simulink model "shelf_cascade"  (R2024b)
settings: Solver=VariableStepAuto  StartTime=0.0  StopTime=10.0  RelTol=1e-3
libraries: dspsrcs4 x1
settings Model: Creator=woutlyen  LastModifiedBy=woutlyen

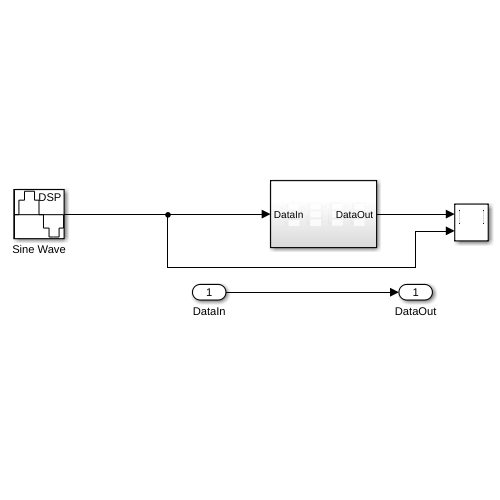
[thumbnail: Simulink's stored preview of the top-level diagram]
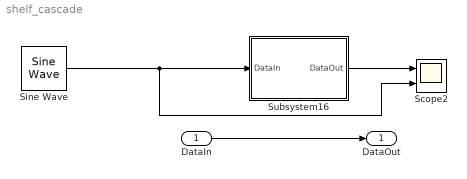
== system shelf_cascade ==
  DataIn : Inport  OutDataTypeStr=fixdt(1,24,23)
  Scope2 : Scope  NumInputPorts=2
  Sine Wave : dspsrcs4/Sine Wave  Amplitude=0.4467  Frequency=12000  Phase=0  SampleMode=Discrete  OutComplex=Real  CompMethod=Table lookup  TableSize=Speed  SampleTime=1/48000  SamplesPerFrame=1  ResetState=Restart at time zero  OutputFrames=off  dataType=Fixed-point  wordLen=24  udDataType=sfix(16)  fracBitsMode=User-defined  numFracBits=23  OutDataTypeStr=fixdt(1,24,23)  LastOutDataTypeStr=fixdt(1,24,23)
  Subsystem16 : Subsystem
  DataOut : Outport
  wires:
  Sine Wave/1 -> Subsystem16/1(DataIn), Scope2/2
  DataIn/1 -> DataOut/1
  Subsystem16/1(DataOut) -> Scope2/1

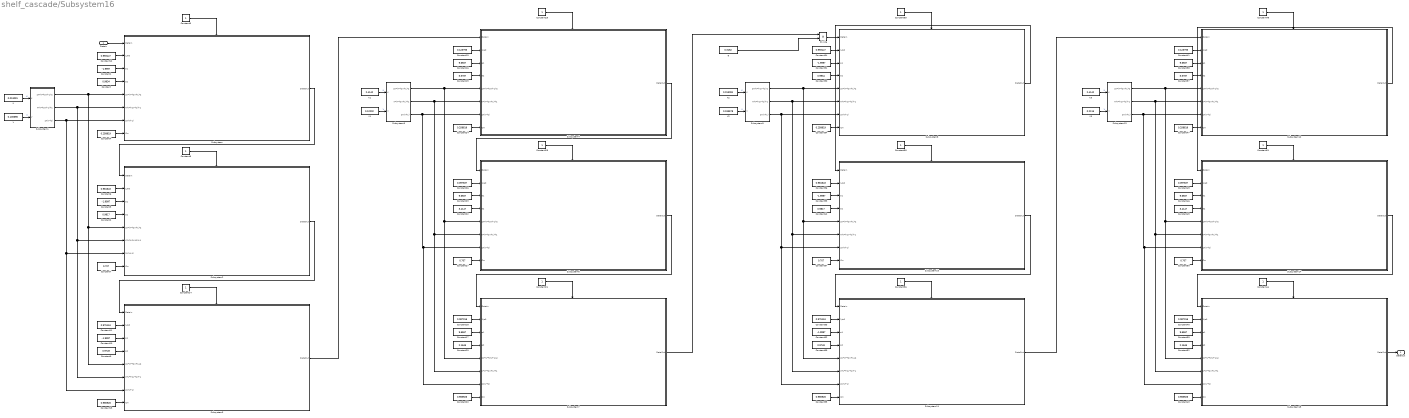
== system shelf_cascade/Subsystem16 ==
  DataIn : Inport
  Constant : Constant  Value=0.9934  OutDataTypeStr=fixdt(1,27,23)
  Constant{1,3,10,31..32,53} (6 alike) : Constant  Value=-1.9997  OutDataTypeStr=fixdt(1,27,23)
  Constant11 : Constant  Value=0.975134  OutDataTypeStr=fixdt(1,27,23)
  Constant12 : Constant  Value=0.993147  OutDataTypeStr=fixdt(1,27,23)
  Constant{13,20,35,43} (4 alike) : Constant  Value=0.965926  OutDataTypeStr=fixdt(1,27,23)
  Constant{5,8,14,21,25,28,36,44,48,51,55,58} (12 alike) : Constant  OutDataTypeStr=boolean
  Constant15 : Constant  Value=5.5787  OutDataTypeStr=fixdt(1,29,23)
  Constant{16..17,23,38..39,46} (6 alike) : Constant  Value=9.6567  OutDataTypeStr=fixdt(1,29,23)
  Constant18 : Constant  Value=0.087016  OutDataTypeStr=fixdt(1,29,23)
  Constant19 : Constant  Value=0.123793  OutDataTypeStr=fixdt(1,29,23)
  Constant2 : Constant  Value=0.9817  OutDataTypeStr=fixdt(1,27,23)
  Constant22 : Constant  Value=3.4147  OutDataTypeStr=fixdt(1,29,23)
  Constant{4,24,47,54} (4 alike) : Constant  Value=0.258819  OutDataTypeStr=fixdt(1,27,23)
  Constant26 : Constant  Value=0.097637  OutDataTypeStr=fixdt(1,29,23)
  Constant{7,27,50,57} (4 alike) : Constant  Value=0.707  OutDataTypeStr=fixdt(1,27,23)
  Constant29 : Constant  Value=2.1645  OutDataTypeStr=fixdt(1,29,23)
  Constant30 : Constant  Value=0.9934  OutDataTypeStr=fixdt(1,27,23)
  Constant33 : Constant  Value=0.975134  OutDataTypeStr=fixdt(1,27,23)
  Constant34 : Constant  Value=0.993147  OutDataTypeStr=fixdt(1,27,23)
  Constant37 : Constant  Value=5.5787  OutDataTypeStr=fixdt(1,29,23)
  Constant40 : Constant  Value=0.087016  OutDataTypeStr=fixdt(1,29,23)
  Constant41 : Constant  Value=0.123793  OutDataTypeStr=fixdt(1,29,23)
  Constant42 : Constant  Value=0.9817  OutDataTypeStr=fixdt(1,27,23)
  Constant45 : Constant  Value=3.4147  OutDataTypeStr=fixdt(1,29,23)
  Constant49 : Constant  Value=0.097637  OutDataTypeStr=fixdt(1,29,23)
  Constant52 : Constant  Value=2.1645  OutDataTypeStr=fixdt(1,29,23)
  Constant56 : Constant  Value=0.981643  OutDataTypeStr=fixdt(1,27,23)
  Constant59 : Constant  Value=0.9749  OutDataTypeStr=fixdt(1,27,23)
  Constant6 : Constant  Value=0.981643  OutDataTypeStr=fixdt(1,27,23)
  Constant9 : Constant  Value=0.9749  OutDataTypeStr=fixdt(1,27,23)
  Divide : Product  Inputs=**  OutDataTypeStr=fixdt(1,27,23)
  K : Constant  Value=0.013091  OutDataTypeStr=fixdt(1,27,23)
  K1 : Constant  Value=2.4142  OutDataTypeStr=fixdt(1,27,23)
  K2 : Constant  Value=0.013091  OutDataTypeStr=fixdt(1,27,23)
  K3 : Constant  Value=2.4142  OutDataTypeStr=fixdt(1,27,23)
  Subsystem : Subsystem
  Subsystem1 : Subsystem
  Subsystem10 : Subsystem
  Subsystem11 : Subsystem
  Subsystem12 : Subsystem
  Subsystem13 : Subsystem
  Subsystem14 : Subsystem
  Subsystem15 : Subsystem
  Subsystem2 : Subsystem
  Subsystem3 : Subsystem
  Subsystem4 : Subsystem
  Subsystem5 : Subsystem
  Subsystem6 : Subsystem
  Subsystem7 : Subsystem
  Subsystem8 : Subsystem
  Subsystem9 : Subsystem
  V : Constant  Value=0.100696  OutDataTypeStr=fixdt(1,27,23)
  V1 : Constant  Value=0.12202  OutDataTypeStr=fixdt(1,27,23)
  V2 : Constant  Value=0.193578  OutDataTypeStr=fixdt(1,27,23)
  V3 : Constant  Value=0.2115  OutDataTypeStr=fixdt(1,27,23)
  g : Constant  Value=0.3162  OutDataTypeStr=fixdt(1,27,23)
  DataOut : Outport
  wires:
  Subsystem2/1(DataOut) -> Subsystem3/1(DataIn)
  Constant7/1 -> Subsystem2/8(Cm)
  Constant21/1 -> Subsystem7/Enable
  Constant5/1 -> Subsystem/Enable
  V/1 -> Subsystem1/2(V)  "V"
  Constant48/1 -> Subsystem12/Enable
  Subsystem4/1(DataOut) -> Subsystem6/1(DataIn)
  Constant22/1 -> Subsystem6/4(a2)
  Constant16/1 -> Subsystem4/3(a1)
  Constant25/1 -> Subsystem4/Enable
  Subsystem7/1(DataOut) -> Divide/1
  Constant12/1 -> Subsystem/2(1/a0)
  V2/1 -> Subsystem9/2(V)  "V"
  g/1 -> Divide/2
  Subsystem12/1(DataOut) -> Subsystem14/1(DataIn)
  Constant53/1 -> Subsystem10/3(a1)
  Constant33/1 -> Subsystem11/2(1/a0)
  Constant28/1 -> Subsystem6/Enable
  Constant24/1 -> Subsystem4/8(Cm)
  Constant46/1 -> Subsystem14/3(a1)
  Constant8/1 -> Subsystem2/Enable
  Constant54/1 -> Subsystem8/8(Cm)
  Constant15/1 -> Subsystem4/4(a2)
  Subsystem5/2(K²(V²+2V+1)+1) -> Subsystem4/6(K²(V²+2V+1)+1), Subsystem7/6(K²(V²+2V+1)+1), Subsystem6/6(K²(V²+2V+1)+1)
  Constant41/1 -> Subsystem12/2(1/a0)
  Constant43/1 -> Subsystem15/8(Cm)
  Constant56/1 -> Subsystem10/2(1/a0)
  Constant30/1 -> Subsystem8/4(a2)
  Subsystem9/3(2K(V+1)) -> Subsystem8/7(2K(V+1)), Subsystem11/7(2K(V+1)), Subsystem10/7(2K(V+1))
  Subsystem9/1(2K²(V²+2V+1)-2) -> Subsystem8/5(2K²(V²+2V+1)-2), Subsystem11/5(2K²(V²+2V+1)-2), Subsystem10/5(2K²(V²+2V+1)-2)
  K3/1 -> Subsystem13/1(K)  "K"
  Constant49/1 -> Subsystem14/2(1/a0)
  K1/1 -> Subsystem5/1(K)  "K"
  Constant26/1 -> Subsystem6/2(1/a0)
  Subsystem9/2(K²(V²+2V+1)+1) -> Subsystem8/6(K²(V²+2V+1)+1), Subsystem11/6(K²(V²+2V+1)+1), Subsystem10/6(K²(V²+2V+1)+1)
  Constant42/1 -> Subsystem10/4(a2)
  Subsystem13/2(K²(V²+2V+1)+1) -> Subsystem12/6(K²(V²+2V+1)+1), Subsystem15/6(K²(V²+2V+1)+1), Subsystem14/6(K²(V²+2V+1)+1)
  Constant39/1 -> Subsystem15/3(a1)
  Constant58/1 -> Subsystem10/Enable
  Constant4/1 -> Subsystem/8(Cm)
  Constant/1 -> Subsystem/4(a2)
  Constant20/1 -> Subsystem7/8(Cm)
  V1/1 -> Subsystem5/2(V)  "V"
  DataIn/1 -> Subsystem/1(DataIn)
  Constant13/1 -> Subsystem3/8(Cm)
  Constant11/1 -> Subsystem3/2(1/a0)
  Constant27/1 -> Subsystem6/8(Cm)
  Subsystem14/1(DataOut) -> Subsystem15/1(DataIn)
  K/1 -> Subsystem1/1(K)  "K"
  Constant18/1 -> Subsystem7/2(1/a0)
  Subsystem1/1(2K²(V²+2V+1)-2) -> Subsystem/5(2K²(V²+2V+1)-2), Subsystem3/5(2K²(V²+2V+1)-2), Subsystem2/5(2K²(V²+2V+1)-2)
  Constant23/1 -> Subsystem6/3(a1)
  Subsystem6/1(DataOut) -> Subsystem7/1(DataIn)
  K2/1 -> Subsystem9/1(K)  "K"
  Constant50/1 -> Subsystem14/8(Cm)
  Constant2/1 -> Subsystem2/4(a2)
  Subsystem11/1(DataOut) -> Subsystem12/1(DataIn)
  V3/1 -> Subsystem13/2(V)  "V"
  Constant29/1 -> Subsystem7/4(a2)
  Constant1/1 -> Subsystem/3(a1)
  Subsystem5/3(2K(V+1)) -> Subsystem4/7(2K(V+1)), Subsystem7/7(2K(V+1)), Subsystem6/7(2K(V+1))
  Subsystem1/3(2K(V+1)) -> Subsystem/7(2K(V+1)), Subsystem3/7(2K(V+1)), Subsystem2/7(2K(V+1))
  Constant57/1 -> Subsystem10/8(Cm)
  Constant14/1 -> Subsystem3/Enable
  Subsystem10/1(DataOut) -> Subsystem11/1(DataIn)
  Subsystem/1(DataOut) -> Subsystem2/1(DataIn)
  Constant45/1 -> Subsystem14/4(a2)
  Constant9/1 -> Subsystem3/4(a2)
  Constant35/1 -> Subsystem11/8(Cm)
  Constant17/1 -> Subsystem7/3(a1)
  Constant34/1 -> Subsystem8/2(1/a0)
  Subsystem5/1(2K²(V²+2V+1)-2) -> Subsystem4/5(2K²(V²+2V+1)-2), Subsystem7/5(2K²(V²+2V+1)-2), Subsystem6/5(2K²(V²+2V+1)-2)
  Constant6/1 -> Subsystem2/2(1/a0)
  Subsystem8/1(DataOut) -> Subsystem10/1(DataIn)
  Constant32/1 -> Subsystem11/3(a1)
  Constant59/1 -> Subsystem11/4(a2)
  Constant37/1 -> Subsystem12/4(a2)
  Subsystem3/1(DataOut) -> Subsystem4/1(DataIn)
  Divide/1 -> Subsystem8/1(DataIn)
  Constant52/1 -> Subsystem15/4(a2)
  Constant40/1 -> Subsystem15/2(1/a0)
  Constant3/1 -> Subsystem2/3(a1)
  Constant19/1 -> Subsystem4/2(1/a0)
  Constant55/1 -> Subsystem8/Enable
  Subsystem15/1(DataOut) -> DataOut/1
  Subsystem13/3(2K(V+1)) -> Subsystem12/7(2K(V+1)), Subsystem15/7(2K(V+1)), Subsystem14/7(2K(V+1))
  Constant38/1 -> Subsystem12/3(a1)
  Constant36/1 -> Subsystem11/Enable
  Constant31/1 -> Subsystem8/3(a1)
  Constant10/1 -> Subsystem3/3(a1)
  Constant47/1 -> Subsystem12/8(Cm)
  Subsystem1/2(K²(V²+2V+1)+1) -> Subsystem/6(K²(V²+2V+1)+1), Subsystem3/6(K²(V²+2V+1)+1), Subsystem2/6(K²(V²+2V+1)+1)
  Constant44/1 -> Subsystem15/Enable
  Constant51/1 -> Subsystem14/Enable
  Subsystem13/1(2K²(V²+2V+1)-2) -> Subsystem12/5(2K²(V²+2V+1)-2), Subsystem15/5(2K²(V²+2V+1)-2), Subsystem14/5(2K²(V²+2V+1)-2)

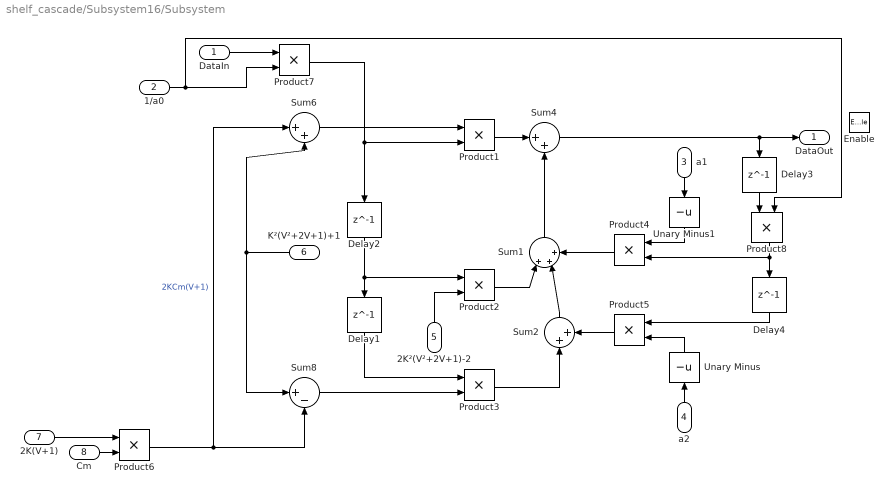
== system shelf_cascade/Subsystem16/Subsystem ==
  DataIn : Inport
  1/a0 : Inport  Port=2
  a1 : Inport  Port=3
  a2 : Inport  Port=4
  2K²(V²+2V+1)-2 : Inport  Port=5
  K²(V²+2V+1)+1 : Inport  Port=6
  2K(V+1) : Inport  Port=7
  Cm : Inport  Port=8
  Enable : EnablePort
  Delay{1..4} (4 alike) : Delay  DelayLength=1  InitialCondition=0
  Product{1..8} (8 alike) : Product  OutDataTypeStr=fixdt(1,27,23)
  Sum1 : Sum  Inputs=|+++
  Sum2 : Sum  Inputs=|++
  Sum4 : Sum  Inputs=|++
  Sum6 : Sum  Inputs=|++
  Sum8 : Sum  Inputs=|+-
  Unary Minus : UnaryMinus
  Unary Minus1 : UnaryMinus
  DataOut : Outport  VectorParamsAs1DForOutWhenUnconnected=off
  wires:
  Sum1/1 -> Sum4/2
  Product5/1 -> Sum2/2
  a1/1 -> Unary Minus1/1
  Unary Minus1/1 -> Product4/1
  Delay3/1 -> Product8/1
  DataIn/1 -> Product7/1
  Product3/1 -> Sum2/1
  1/a0/1 -> Product8/2, Product7/2
  K²(V²+2V+1)+1/1 -> Sum8/1, Sum6/2
  Unary Minus/1 -> Product5/2
  2K(V+1)/1 -> Product6/1
  Sum4/1 -> DataOut/1, Delay3/1
  Delay4/1 -> Product5/1
  Sum6/1 -> Product1/1
  2K²(V²+2V+1)-2/1 -> Product2/2
  Sum8/1 -> Product3/2
  Product6/1 -> Sum6/1, Sum8/2  "2KCm(V+1)"
  Product8/1 -> Product4/2, Delay4/1
  Product2/1 -> Sum1/1
  Product4/1 -> Sum1/3
  Delay1/1 -> Product3/1
  Delay2/1 -> Product2/1, Delay1/1
  a2/1 -> Unary Minus/1
  Sum2/1 -> Sum1/2
  Product7/1 -> Product1/2, Delay2/1
  Cm/1 -> Product6/2
  Product1/1 -> Sum4/1

== system shelf_cascade/Subsystem16/Subsystem1 ==
  K : Inport
  V : Inport  Port=2
  Constant10 : Constant  OutDataTypeStr=fixdt(1,27,23)  SampleTime=-1
  Constant{6,8,11,13} (4 alike) : Constant  Value=2  OutDataTypeStr=fixdt(1,27,23)  SampleTime=-1
  Constant7 : Constant  OutDataTypeStr=fixdt(1,27,23)  SampleTime=-1
  Constant9 : Constant  OutDataTypeStr=fixdt(1,27,23)  SampleTime=-1
  Product{,6..11} (7 alike) : Product  OutDataTypeStr=fixdt(1,27,23)
  Sum3 : Sum  Inputs=|++
  Sum5 : Sum  Inputs=|+++
  Sum6 : Sum  Inputs=|++
  Sum7 : Sum  Inputs=|+-
  2K²(V²+2V+1)-2 : Outport
  K²(V²+2V+1)+1 : Outport  Port=2
  2K(V+1) : Outport  Port=3
  wires:
  Constant8/1 -> Product9/2
  Product11/1 -> Sum7/1  "2K²(V²+2V+1)"
  Constant7/1 -> Sum3/1
  Constant10/1 -> Sum6/2
  Sum3/1 -> Product7/2  "V+1"
  Constant9/1 -> Sum5/3
  Sum6/1 -> K²(V²+2V+1)+1/1  "K²(V²+2V+1)+1"
  Product10/1 -> Sum6/1, Product11/1  "K²(V²+2V+1)"
  Sum5/1 -> Product10/2  "V²+2V+1"
  Constant11/1 -> Sum7/2
  Product6/1 -> Product7/1  "2K"
  Product7/1 -> 2K(V+1)/1  "2K(V+1)"
  V/1 -> Product9/1, Product8/2, Product8/1, Sum3/2  "V"
  Sum7/1 -> 2K²(V²+2V+1)-2/1  "2K²(V²+2V+1)-2"
  K/1 -> Product6/1, Product/2, Product/1  "K"
  Constant6/1 -> Product6/2
  Product8/1 -> Sum5/1  "V²"
  Constant13/1 -> Product11/2
  Product9/1 -> Sum5/2  "2V"
  Product/1 -> Product10/1  "K²"

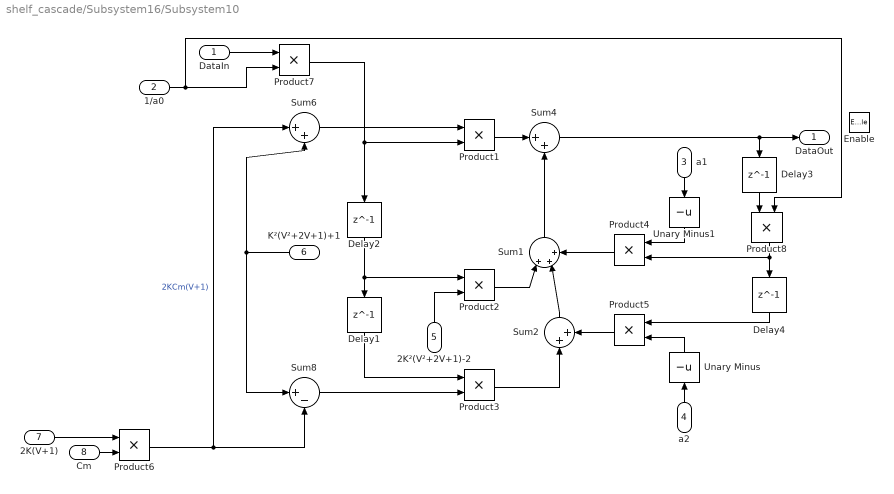
== system shelf_cascade/Subsystem16/Subsystem10 ==
  DataIn : Inport
  1/a0 : Inport  Port=2
  a1 : Inport  Port=3
  a2 : Inport  Port=4
  2K²(V²+2V+1)-2 : Inport  Port=5
  K²(V²+2V+1)+1 : Inport  Port=6
  2K(V+1) : Inport  Port=7
  Cm : Inport  Port=8
  Enable : EnablePort
  Delay{1..4} (4 alike) : Delay  DelayLength=1  InitialCondition=0
  Product{1..8} (8 alike) : Product  OutDataTypeStr=fixdt(1,27,23)
  Sum1 : Sum  Inputs=|+++
  Sum2 : Sum  Inputs=|++
  Sum4 : Sum  Inputs=|++
  Sum6 : Sum  Inputs=|++
  Sum8 : Sum  Inputs=|+-
  Unary Minus : UnaryMinus
  Unary Minus1 : UnaryMinus
  DataOut : Outport  VectorParamsAs1DForOutWhenUnconnected=off
  wires:
  K²(V²+2V+1)+1/1 -> Sum8/1, Sum6/2
  Product1/1 -> Sum4/1
  Cm/1 -> Product6/2
  Sum1/1 -> Sum4/2
  Delay2/1 -> Product2/1, Delay1/1
  Delay1/1 -> Product3/1
  2K(V+1)/1 -> Product6/1
  Product8/1 -> Product4/2, Delay4/1
  Sum6/1 -> Product1/1
  Product6/1 -> Sum6/1, Sum8/2  "2KCm(V+1)"
  Product7/1 -> Product1/2, Delay2/1
  Unary Minus1/1 -> Product4/1
  2K²(V²+2V+1)-2/1 -> Product2/2
  Unary Minus/1 -> Product5/2
  Sum2/1 -> Sum1/2
  Product4/1 -> Sum1/3
  1/a0/1 -> Product8/2, Product7/2
  Product5/1 -> Sum2/2
  Sum4/1 -> DataOut/1, Delay3/1
  a2/1 -> Unary Minus/1
  Delay3/1 -> Product8/1
  DataIn/1 -> Product7/1
  Product3/1 -> Sum2/1
  Product2/1 -> Sum1/1
  Sum8/1 -> Product3/2
  a1/1 -> Unary Minus1/1
  Delay4/1 -> Product5/1

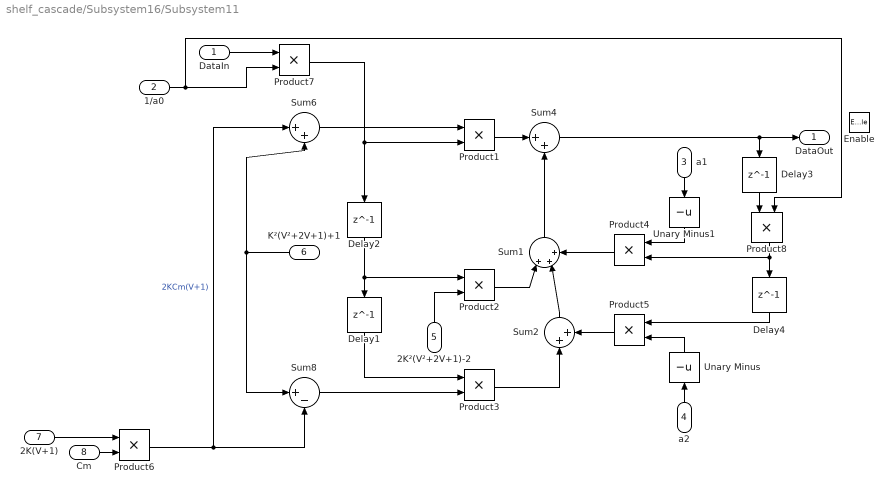
== system shelf_cascade/Subsystem16/Subsystem11 ==
  DataIn : Inport
  1/a0 : Inport  Port=2
  a1 : Inport  Port=3
  a2 : Inport  Port=4
  2K²(V²+2V+1)-2 : Inport  Port=5
  K²(V²+2V+1)+1 : Inport  Port=6
  2K(V+1) : Inport  Port=7
  Cm : Inport  Port=8
  Enable : EnablePort
  Delay{1..4} (4 alike) : Delay  DelayLength=1  InitialCondition=0
  Product{1..8} (8 alike) : Product  OutDataTypeStr=fixdt(1,27,23)
  Sum1 : Sum  Inputs=|+++
  Sum2 : Sum  Inputs=|++
  Sum4 : Sum  Inputs=|++
  Sum6 : Sum  Inputs=|++
  Sum8 : Sum  Inputs=|+-
  Unary Minus : UnaryMinus
  Unary Minus1 : UnaryMinus
  DataOut : Outport  VectorParamsAs1DForOutWhenUnconnected=off
  wires:
  K²(V²+2V+1)+1/1 -> Sum8/1, Sum6/2
  Product1/1 -> Sum4/1
  Cm/1 -> Product6/2
  Sum1/1 -> Sum4/2
  Delay2/1 -> Product2/1, Delay1/1
  Delay1/1 -> Product3/1
  2K(V+1)/1 -> Product6/1
  Product8/1 -> Product4/2, Delay4/1
  Sum6/1 -> Product1/1
  Product6/1 -> Sum6/1, Sum8/2  "2KCm(V+1)"
  Product7/1 -> Product1/2, Delay2/1
  Unary Minus1/1 -> Product4/1
  2K²(V²+2V+1)-2/1 -> Product2/2
  Unary Minus/1 -> Product5/2
  Sum2/1 -> Sum1/2
  Product4/1 -> Sum1/3
  1/a0/1 -> Product8/2, Product7/2
  Product5/1 -> Sum2/2
  Sum4/1 -> DataOut/1, Delay3/1
  a2/1 -> Unary Minus/1
  Delay3/1 -> Product8/1
  DataIn/1 -> Product7/1
  Product3/1 -> Sum2/1
  Product2/1 -> Sum1/1
  Sum8/1 -> Product3/2
  a1/1 -> Unary Minus1/1
  Delay4/1 -> Product5/1

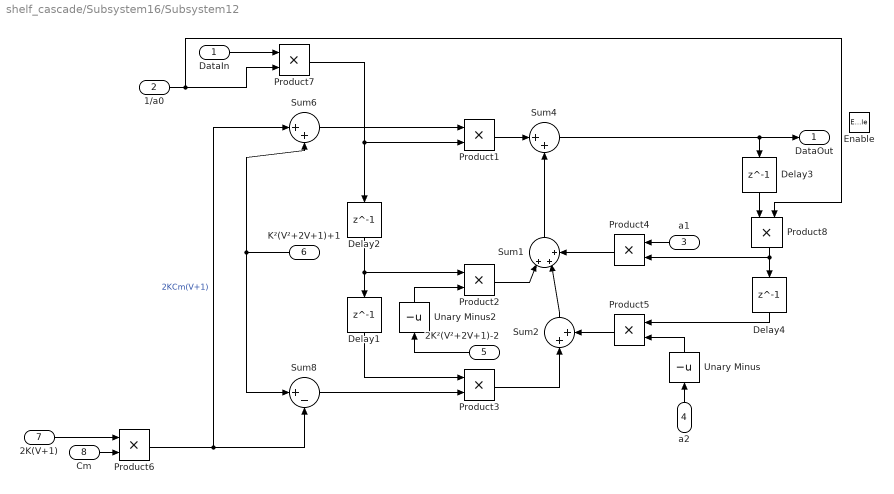
== system shelf_cascade/Subsystem16/Subsystem12 ==
  DataIn : Inport
  1/a0 : Inport  Port=2
  a1 : Inport  Port=3
  a2 : Inport  Port=4
  2K²(V²+2V+1)-2 : Inport  Port=5
  K²(V²+2V+1)+1 : Inport  Port=6
  2K(V+1) : Inport  Port=7
  Cm : Inport  Port=8
  Enable : EnablePort
  Delay{1..4} (4 alike) : Delay  DelayLength=1  InitialCondition=0
  Product{1..5,7..8} (7 alike) : Product  OutDataTypeStr=fixdt(1,27,23)
  Product6 : Product  OutDataTypeStr=fixdt(1,29,23)
  Sum1 : Sum  Inputs=|+++
  Sum2 : Sum  Inputs=|++
  Sum4 : Sum  Inputs=|++
  Sum6 : Sum  Inputs=|++
  Sum8 : Sum  Inputs=|+-
  Unary Minus : UnaryMinus
  Unary Minus2 : UnaryMinus
  DataOut : Outport  VectorParamsAs1DForOutWhenUnconnected=off
  wires:
  Product1/1 -> Sum4/1
  Delay4/1 -> Product5/1
  Delay2/1 -> Delay1/1, Product2/1
  Product4/1 -> Sum1/3
  DataIn/1 -> Product7/1
  Delay1/1 -> Product3/1
  Sum1/1 -> Sum4/2
  Unary Minus2/1 -> Product2/2
  Product2/1 -> Sum1/1
  Product3/1 -> Sum2/1
  Cm/1 -> Product6/2
  Unary Minus/1 -> Product5/2
  Product6/1 -> Sum6/1, Sum8/2  "2KCm(V+1)"
  Sum4/1 -> DataOut/1, Delay3/1
  Sum6/1 -> Product1/1
  2K²(V²+2V+1)-2/1 -> Unary Minus2/1
  1/a0/1 -> Product8/2, Product7/2
  Sum2/1 -> Sum1/2
  a1/1 -> Product4/1
  Product8/1 -> Product4/2, Delay4/1
  2K(V+1)/1 -> Product6/1
  a2/1 -> Unary Minus/1
  Sum8/1 -> Product3/2
  Product7/1 -> Product1/2, Delay2/1
  K²(V²+2V+1)+1/1 -> Sum8/1, Sum6/2
  Product5/1 -> Sum2/2
  Delay3/1 -> Product8/1

== system shelf_cascade/Subsystem16/Subsystem13 ==
  K : Inport
  V : Inport  Port=2
  Constant10 : Constant  OutDataTypeStr=fixdt(1,27,23)  SampleTime=-1
  Constant{6,8,11,13} (4 alike) : Constant  Value=2  OutDataTypeStr=fixdt(1,27,23)  SampleTime=-1
  Constant7 : Constant  OutDataTypeStr=fixdt(1,27,23)  SampleTime=-1
  Constant9 : Constant  OutDataTypeStr=fixdt(1,27,23)  SampleTime=-1
  Product{,6..11} (7 alike) : Product  OutDataTypeStr=fixdt(1,29,23)
  Sum3 : Sum  Inputs=|++
  Sum5 : Sum  Inputs=|+++
  Sum6 : Sum  Inputs=|++
  Sum7 : Sum  Inputs=|+-
  2K²(V²+2V+1)-2 : Outport
  K²(V²+2V+1)+1 : Outport  Port=2
  2K(V+1) : Outport  Port=3
  wires:
  Product8/1 -> Sum5/1  "V²"
  Sum6/1 -> K²(V²+2V+1)+1/1  "K²(V²+2V+1)+1"
  Product9/1 -> Sum5/2  "2V"
  Constant13/1 -> Product11/2
  Constant10/1 -> Sum6/2
  Product11/1 -> Sum7/1  "2K²(V²+2V+1)"
  Product/1 -> Product10/1  "K²"
  Constant7/1 -> Sum3/1
  K/1 -> Product6/1, Product/2, Product/1  "K"
  Sum3/1 -> Product7/2  "V+1"
  Constant8/1 -> Product9/2
  Product6/1 -> Product7/1  "2K"
  Sum7/1 -> 2K²(V²+2V+1)-2/1  "2K²(V²+2V+1)-2"
  Constant9/1 -> Sum5/3
  Constant6/1 -> Product6/2
  Product7/1 -> 2K(V+1)/1  "2K(V+1)"
  V/1 -> Product9/1, Product8/2, Product8/1, Sum3/2  "V"
  Sum5/1 -> Product10/2  "V²+2V+1"
  Constant11/1 -> Sum7/2
  Product10/1 -> Sum6/1, Product11/1  "K²(V²+2V+1)"

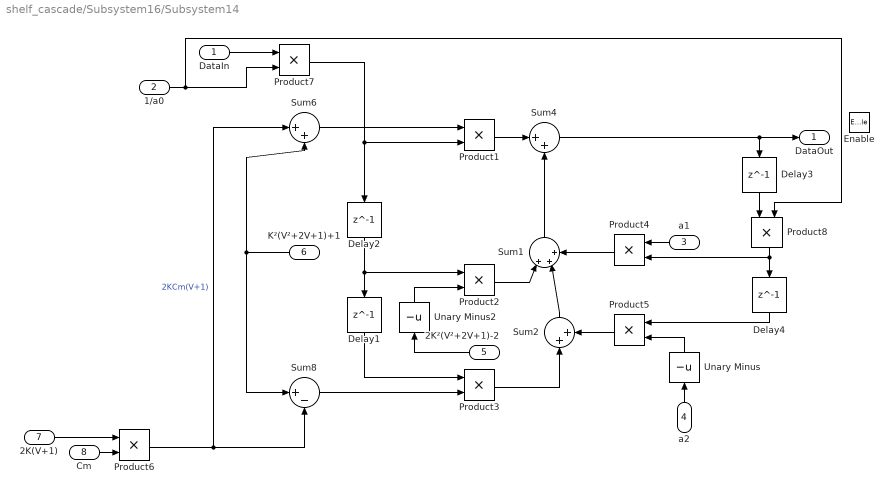
== system shelf_cascade/Subsystem16/Subsystem14 ==
  DataIn : Inport
  1/a0 : Inport  Port=2
  a1 : Inport  Port=3
  a2 : Inport  Port=4
  2K²(V²+2V+1)-2 : Inport  Port=5
  K²(V²+2V+1)+1 : Inport  Port=6
  2K(V+1) : Inport  Port=7
  Cm : Inport  Port=8
  Enable : EnablePort
  Delay{1..4} (4 alike) : Delay  DelayLength=1  InitialCondition=0
  Product{1..5,7..8} (7 alike) : Product  OutDataTypeStr=fixdt(1,27,23)
  Product6 : Product  OutDataTypeStr=fixdt(1,29,23)
  Sum1 : Sum  Inputs=|+++
  Sum2 : Sum  Inputs=|++
  Sum4 : Sum  Inputs=|++
  Sum6 : Sum  Inputs=|++
  Sum8 : Sum  Inputs=|+-
  Unary Minus : UnaryMinus
  Unary Minus2 : UnaryMinus
  DataOut : Outport  VectorParamsAs1DForOutWhenUnconnected=off
  wires:
  Product1/1 -> Sum4/1
  Delay4/1 -> Product5/1
  Delay2/1 -> Delay1/1, Product2/1
  Product4/1 -> Sum1/3
  DataIn/1 -> Product7/1
  Delay1/1 -> Product3/1
  Sum1/1 -> Sum4/2
  Unary Minus2/1 -> Product2/2
  Product2/1 -> Sum1/1
  Product3/1 -> Sum2/1
  Cm/1 -> Product6/2
  Unary Minus/1 -> Product5/2
  Product6/1 -> Sum6/1, Sum8/2  "2KCm(V+1)"
  Sum4/1 -> DataOut/1, Delay3/1
  Sum6/1 -> Product1/1
  2K²(V²+2V+1)-2/1 -> Unary Minus2/1
  1/a0/1 -> Product8/2, Product7/2
  Sum2/1 -> Sum1/2
  a1/1 -> Product4/1
  Product8/1 -> Product4/2, Delay4/1
  2K(V+1)/1 -> Product6/1
  a2/1 -> Unary Minus/1
  Sum8/1 -> Product3/2
  Product7/1 -> Product1/2, Delay2/1
  K²(V²+2V+1)+1/1 -> Sum8/1, Sum6/2
  Product5/1 -> Sum2/2
  Delay3/1 -> Product8/1

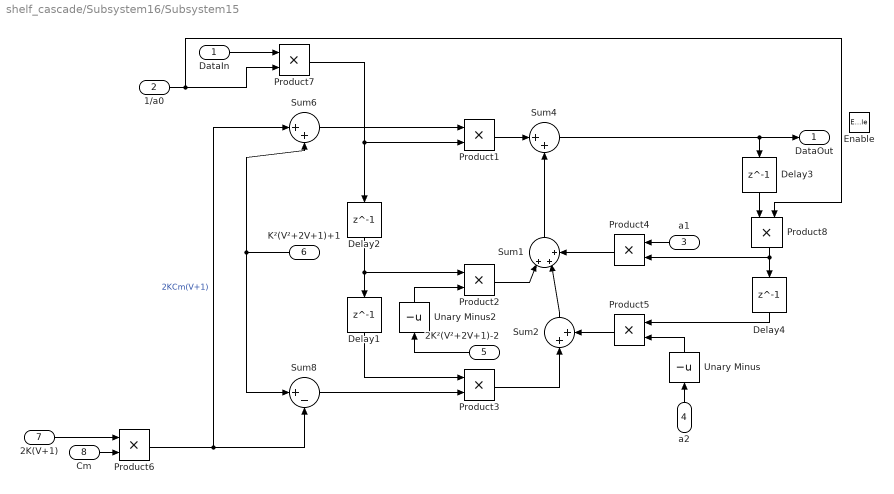
== system shelf_cascade/Subsystem16/Subsystem15 ==
  DataIn : Inport
  1/a0 : Inport  Port=2
  a1 : Inport  Port=3
  a2 : Inport  Port=4
  2K²(V²+2V+1)-2 : Inport  Port=5
  K²(V²+2V+1)+1 : Inport  Port=6
  2K(V+1) : Inport  Port=7
  Cm : Inport  Port=8
  Enable : EnablePort
  Delay{1..4} (4 alike) : Delay  DelayLength=1  InitialCondition=0
  Product{1..5,7..8} (7 alike) : Product  OutDataTypeStr=fixdt(1,27,23)
  Product6 : Product  OutDataTypeStr=fixdt(1,29,23)
  Sum1 : Sum  Inputs=|+++
  Sum2 : Sum  Inputs=|++
  Sum4 : Sum  Inputs=|++
  Sum6 : Sum  Inputs=|++
  Sum8 : Sum  Inputs=|+-
  Unary Minus : UnaryMinus
  Unary Minus2 : UnaryMinus
  DataOut : Outport  VectorParamsAs1DForOutWhenUnconnected=off
  wires:
  Product1/1 -> Sum4/1
  Delay4/1 -> Product5/1
  Delay2/1 -> Delay1/1, Product2/1
  Product4/1 -> Sum1/3
  DataIn/1 -> Product7/1
  Delay1/1 -> Product3/1
  Sum1/1 -> Sum4/2
  Unary Minus2/1 -> Product2/2
  Product2/1 -> Sum1/1
  Product3/1 -> Sum2/1
  Cm/1 -> Product6/2
  Unary Minus/1 -> Product5/2
  Product6/1 -> Sum6/1, Sum8/2  "2KCm(V+1)"
  Sum4/1 -> DataOut/1, Delay3/1
  Sum6/1 -> Product1/1
  2K²(V²+2V+1)-2/1 -> Unary Minus2/1
  1/a0/1 -> Product8/2, Product7/2
  Sum2/1 -> Sum1/2
  a1/1 -> Product4/1
  Product8/1 -> Product4/2, Delay4/1
  2K(V+1)/1 -> Product6/1
  a2/1 -> Unary Minus/1
  Sum8/1 -> Product3/2
  Product7/1 -> Product1/2, Delay2/1
  K²(V²+2V+1)+1/1 -> Sum8/1, Sum6/2
  Product5/1 -> Sum2/2
  Delay3/1 -> Product8/1

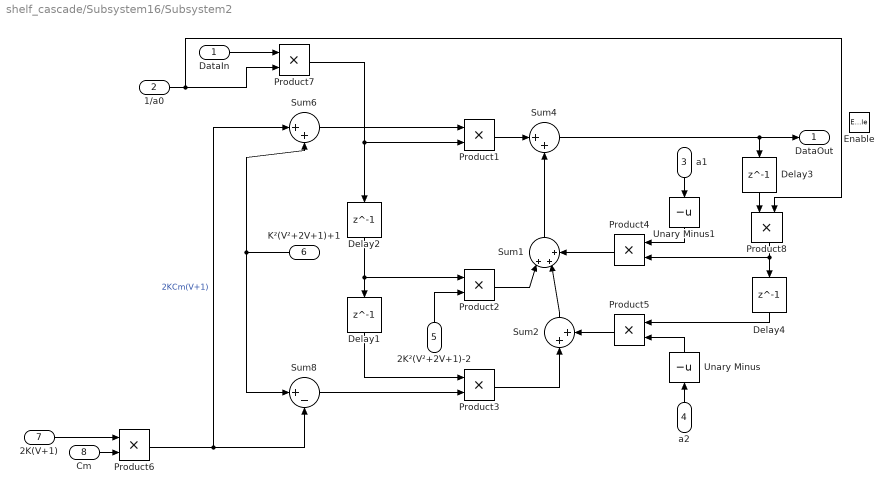
== system shelf_cascade/Subsystem16/Subsystem2 ==
  DataIn : Inport
  1/a0 : Inport  Port=2
  a1 : Inport  Port=3
  a2 : Inport  Port=4
  2K²(V²+2V+1)-2 : Inport  Port=5
  K²(V²+2V+1)+1 : Inport  Port=6
  2K(V+1) : Inport  Port=7
  Cm : Inport  Port=8
  Enable : EnablePort
  Delay{1..4} (4 alike) : Delay  DelayLength=1  InitialCondition=0
  Product{1..8} (8 alike) : Product  OutDataTypeStr=fixdt(1,27,23)
  Sum1 : Sum  Inputs=|+++
  Sum2 : Sum  Inputs=|++
  Sum4 : Sum  Inputs=|++
  Sum6 : Sum  Inputs=|++
  Sum8 : Sum  Inputs=|+-
  Unary Minus : UnaryMinus
  Unary Minus1 : UnaryMinus
  DataOut : Outport  VectorParamsAs1DForOutWhenUnconnected=off
  wires:
  K²(V²+2V+1)+1/1 -> Sum8/1, Sum6/2
  Product1/1 -> Sum4/1
  Cm/1 -> Product6/2
  Sum1/1 -> Sum4/2
  Delay2/1 -> Product2/1, Delay1/1
  Delay1/1 -> Product3/1
  2K(V+1)/1 -> Product6/1
  Product8/1 -> Product4/2, Delay4/1
  Sum6/1 -> Product1/1
  Product6/1 -> Sum6/1, Sum8/2  "2KCm(V+1)"
  Product7/1 -> Product1/2, Delay2/1
  Unary Minus1/1 -> Product4/1
  2K²(V²+2V+1)-2/1 -> Product2/2
  Unary Minus/1 -> Product5/2
  Sum2/1 -> Sum1/2
  Product4/1 -> Sum1/3
  1/a0/1 -> Product8/2, Product7/2
  Product5/1 -> Sum2/2
  Sum4/1 -> DataOut/1, Delay3/1
  a2/1 -> Unary Minus/1
  Delay3/1 -> Product8/1
  DataIn/1 -> Product7/1
  Product3/1 -> Sum2/1
  Product2/1 -> Sum1/1
  Sum8/1 -> Product3/2
  a1/1 -> Unary Minus1/1
  Delay4/1 -> Product5/1

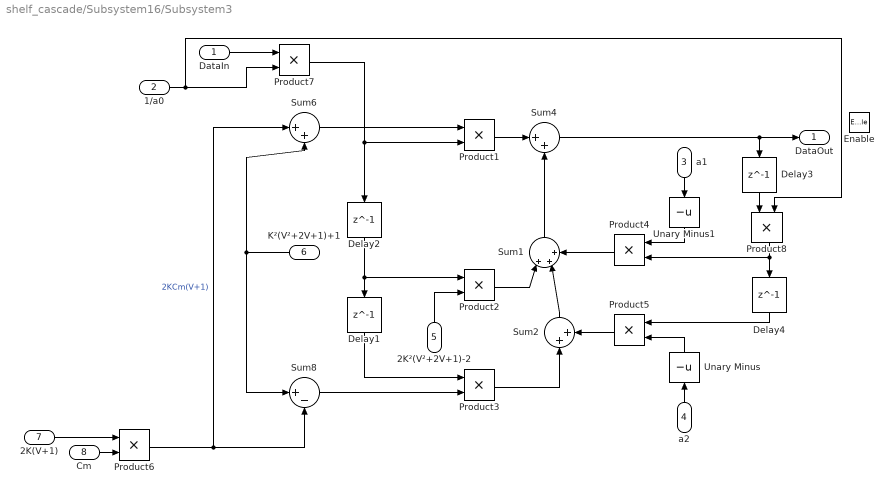
== system shelf_cascade/Subsystem16/Subsystem3 ==
  DataIn : Inport
  1/a0 : Inport  Port=2
  a1 : Inport  Port=3
  a2 : Inport  Port=4
  2K²(V²+2V+1)-2 : Inport  Port=5
  K²(V²+2V+1)+1 : Inport  Port=6
  2K(V+1) : Inport  Port=7
  Cm : Inport  Port=8
  Enable : EnablePort
  Delay{1..4} (4 alike) : Delay  DelayLength=1  InitialCondition=0
  Product{1..8} (8 alike) : Product  OutDataTypeStr=fixdt(1,27,23)
  Sum1 : Sum  Inputs=|+++
  Sum2 : Sum  Inputs=|++
  Sum4 : Sum  Inputs=|++
  Sum6 : Sum  Inputs=|++
  Sum8 : Sum  Inputs=|+-
  Unary Minus : UnaryMinus
  Unary Minus1 : UnaryMinus
  DataOut : Outport  VectorParamsAs1DForOutWhenUnconnected=off
  wires:
  K²(V²+2V+1)+1/1 -> Sum8/1, Sum6/2
  Product1/1 -> Sum4/1
  Cm/1 -> Product6/2
  Sum1/1 -> Sum4/2
  Delay2/1 -> Product2/1, Delay1/1
  Delay1/1 -> Product3/1
  2K(V+1)/1 -> Product6/1
  Product8/1 -> Product4/2, Delay4/1
  Sum6/1 -> Product1/1
  Product6/1 -> Sum6/1, Sum8/2  "2KCm(V+1)"
  Product7/1 -> Product1/2, Delay2/1
  Unary Minus1/1 -> Product4/1
  2K²(V²+2V+1)-2/1 -> Product2/2
  Unary Minus/1 -> Product5/2
  Sum2/1 -> Sum1/2
  Product4/1 -> Sum1/3
  1/a0/1 -> Product8/2, Product7/2
  Product5/1 -> Sum2/2
  Sum4/1 -> DataOut/1, Delay3/1
  a2/1 -> Unary Minus/1
  Delay3/1 -> Product8/1
  DataIn/1 -> Product7/1
  Product3/1 -> Sum2/1
  Product2/1 -> Sum1/1
  Sum8/1 -> Product3/2
  a1/1 -> Unary Minus1/1
  Delay4/1 -> Product5/1

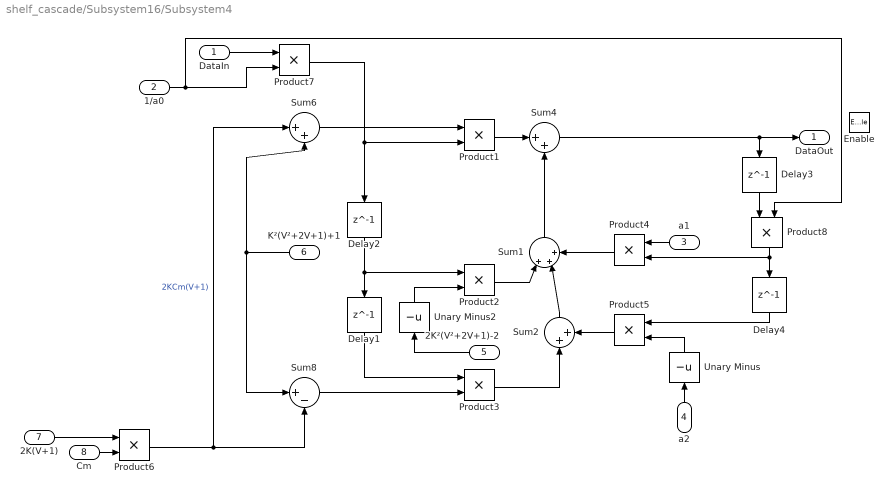
== system shelf_cascade/Subsystem16/Subsystem4 ==
  DataIn : Inport
  1/a0 : Inport  Port=2
  a1 : Inport  Port=3
  a2 : Inport  Port=4
  2K²(V²+2V+1)-2 : Inport  Port=5
  K²(V²+2V+1)+1 : Inport  Port=6
  2K(V+1) : Inport  Port=7
  Cm : Inport  Port=8
  Enable : EnablePort
  Delay{1..4} (4 alike) : Delay  DelayLength=1  InitialCondition=0
  Product{1..5,7..8} (7 alike) : Product  OutDataTypeStr=fixdt(1,27,23)
  Product6 : Product  OutDataTypeStr=fixdt(1,29,23)
  Sum1 : Sum  Inputs=|+++
  Sum2 : Sum  Inputs=|++
  Sum4 : Sum  Inputs=|++
  Sum6 : Sum  Inputs=|++
  Sum8 : Sum  Inputs=|+-
  Unary Minus : UnaryMinus
  Unary Minus2 : UnaryMinus
  DataOut : Outport  VectorParamsAs1DForOutWhenUnconnected=off
  wires:
  Sum1/1 -> Sum4/2
  Product5/1 -> Sum2/2
  a1/1 -> Product4/1
  Delay3/1 -> Product8/1
  DataIn/1 -> Product7/1
  Product3/1 -> Sum2/1
  1/a0/1 -> Product8/2, Product7/2
  K²(V²+2V+1)+1/1 -> Sum8/1, Sum6/2
  Unary Minus/1 -> Product5/2
  2K(V+1)/1 -> Product6/1
  Sum4/1 -> DataOut/1, Delay3/1
  Delay4/1 -> Product5/1
  Sum6/1 -> Product1/1
  2K²(V²+2V+1)-2/1 -> Unary Minus2/1
  Sum8/1 -> Product3/2
  Product6/1 -> Sum6/1, Sum8/2  "2KCm(V+1)"
  Product8/1 -> Product4/2, Delay4/1
  Product2/1 -> Sum1/1
  Product4/1 -> Sum1/3
  Delay1/1 -> Product3/1
  Delay2/1 -> Delay1/1, Product2/1
  a2/1 -> Unary Minus/1
  Sum2/1 -> Sum1/2
  Product7/1 -> Product1/2, Delay2/1
  Cm/1 -> Product6/2
  Product1/1 -> Sum4/1
  Unary Minus2/1 -> Product2/2

== system shelf_cascade/Subsystem16/Subsystem5 ==
  K : Inport
  V : Inport  Port=2
  Constant10 : Constant  OutDataTypeStr=fixdt(1,27,23)  SampleTime=-1
  Constant{6,8,11,13} (4 alike) : Constant  Value=2  OutDataTypeStr=fixdt(1,27,23)  SampleTime=-1
  Constant7 : Constant  OutDataTypeStr=fixdt(1,27,23)  SampleTime=-1
  Constant9 : Constant  OutDataTypeStr=fixdt(1,27,23)  SampleTime=-1
  Product{,6..11} (7 alike) : Product  OutDataTypeStr=fixdt(1,29,23)
  Sum3 : Sum  Inputs=|++
  Sum5 : Sum  Inputs=|+++
  Sum6 : Sum  Inputs=|++
  Sum7 : Sum  Inputs=|+-
  2K²(V²+2V+1)-2 : Outport
  K²(V²+2V+1)+1 : Outport  Port=2
  2K(V+1) : Outport  Port=3
  wires:
  Sum7/1 -> 2K²(V²+2V+1)-2/1  "2K²(V²+2V+1)-2"
  K/1 -> Product6/1, Product/2, Product/1  "K"
  Product6/1 -> Product7/1  "2K"
  Product10/1 -> Sum6/1, Product11/1  "K²(V²+2V+1)"
  Product11/1 -> Sum7/1  "2K²(V²+2V+1)"
  Constant7/1 -> Sum3/1
  Constant11/1 -> Sum7/2
  Sum3/1 -> Product7/2  "V+1"
  Product7/1 -> 2K(V+1)/1  "2K(V+1)"
  Constant10/1 -> Sum6/2
  V/1 -> Product9/1, Product8/2, Product8/1, Sum3/2  "V"
  Constant9/1 -> Sum5/3
  Product/1 -> Product10/1  "K²"
  Sum6/1 -> K²(V²+2V+1)+1/1  "K²(V²+2V+1)+1"
  Constant13/1 -> Product11/2
  Product8/1 -> Sum5/1  "V²"
  Constant6/1 -> Product6/2
  Product9/1 -> Sum5/2  "2V"
  Sum5/1 -> Product10/2  "V²+2V+1"
  Constant8/1 -> Product9/2

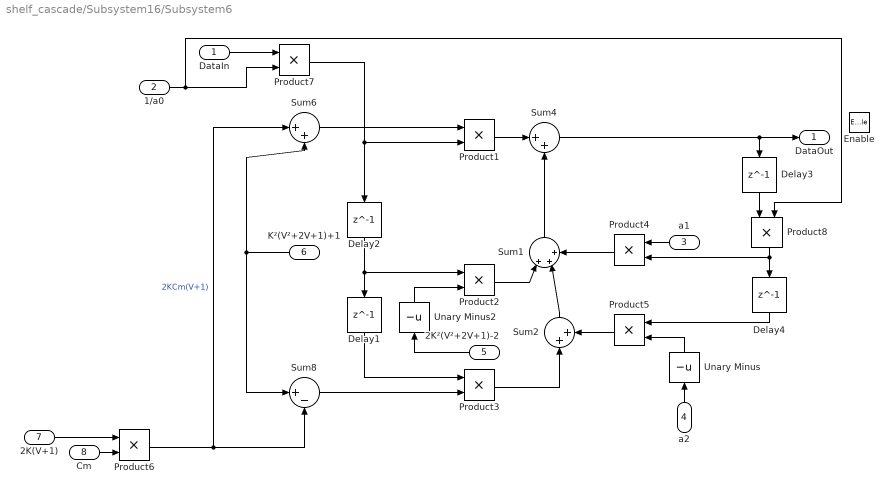
== system shelf_cascade/Subsystem16/Subsystem6 ==
  DataIn : Inport
  1/a0 : Inport  Port=2
  a1 : Inport  Port=3
  a2 : Inport  Port=4
  2K²(V²+2V+1)-2 : Inport  Port=5
  K²(V²+2V+1)+1 : Inport  Port=6
  2K(V+1) : Inport  Port=7
  Cm : Inport  Port=8
  Enable : EnablePort
  Delay{1..4} (4 alike) : Delay  DelayLength=1  InitialCondition=0
  Product{1..5,7..8} (7 alike) : Product  OutDataTypeStr=fixdt(1,27,23)
  Product6 : Product  OutDataTypeStr=fixdt(1,29,23)
  Sum1 : Sum  Inputs=|+++
  Sum2 : Sum  Inputs=|++
  Sum4 : Sum  Inputs=|++
  Sum6 : Sum  Inputs=|++
  Sum8 : Sum  Inputs=|+-
  Unary Minus : UnaryMinus
  Unary Minus2 : UnaryMinus
  DataOut : Outport  VectorParamsAs1DForOutWhenUnconnected=off
  wires:
  Product1/1 -> Sum4/1
  Delay4/1 -> Product5/1
  Delay2/1 -> Delay1/1, Product2/1
  Product4/1 -> Sum1/3
  DataIn/1 -> Product7/1
  Delay1/1 -> Product3/1
  Sum1/1 -> Sum4/2
  Unary Minus2/1 -> Product2/2
  Product2/1 -> Sum1/1
  Product3/1 -> Sum2/1
  Cm/1 -> Product6/2
  Unary Minus/1 -> Product5/2
  Product6/1 -> Sum6/1, Sum8/2  "2KCm(V+1)"
  Sum4/1 -> DataOut/1, Delay3/1
  Sum6/1 -> Product1/1
  2K²(V²+2V+1)-2/1 -> Unary Minus2/1
  1/a0/1 -> Product8/2, Product7/2
  Sum2/1 -> Sum1/2
  a1/1 -> Product4/1
  Product8/1 -> Product4/2, Delay4/1
  2K(V+1)/1 -> Product6/1
  a2/1 -> Unary Minus/1
  Sum8/1 -> Product3/2
  Product7/1 -> Product1/2, Delay2/1
  K²(V²+2V+1)+1/1 -> Sum8/1, Sum6/2
  Product5/1 -> Sum2/2
  Delay3/1 -> Product8/1

== system shelf_cascade/Subsystem16/Subsystem7 ==
  DataIn : Inport
  1/a0 : Inport  Port=2
  a1 : Inport  Port=3
  a2 : Inport  Port=4
  2K²(V²+2V+1)-2 : Inport  Port=5
  K²(V²+2V+1)+1 : Inport  Port=6
  2K(V+1) : Inport  Port=7
  Cm : Inport  Port=8
  Enable : EnablePort
  Delay{1..4} (4 alike) : Delay  DelayLength=1  InitialCondition=0
  Product{1..5,7..8} (7 alike) : Product  OutDataTypeStr=fixdt(1,27,23)
  Product6 : Product  OutDataTypeStr=fixdt(1,29,23)
  Sum1 : Sum  Inputs=|+++
  Sum2 : Sum  Inputs=|++
  Sum4 : Sum  Inputs=|++
  Sum6 : Sum  Inputs=|++
  Sum8 : Sum  Inputs=|+-
  Unary Minus : UnaryMinus
  Unary Minus2 : UnaryMinus
  DataOut : Outport  VectorParamsAs1DForOutWhenUnconnected=off
  wires:
  Product1/1 -> Sum4/1
  Delay4/1 -> Product5/1
  Delay2/1 -> Delay1/1, Product2/1
  Product4/1 -> Sum1/3
  DataIn/1 -> Product7/1
  Delay1/1 -> Product3/1
  Sum1/1 -> Sum4/2
  Unary Minus2/1 -> Product2/2
  Product2/1 -> Sum1/1
  Product3/1 -> Sum2/1
  Cm/1 -> Product6/2
  Unary Minus/1 -> Product5/2
  Product6/1 -> Sum6/1, Sum8/2  "2KCm(V+1)"
  Sum4/1 -> DataOut/1, Delay3/1
  Sum6/1 -> Product1/1
  2K²(V²+2V+1)-2/1 -> Unary Minus2/1
  1/a0/1 -> Product8/2, Product7/2
  Sum2/1 -> Sum1/2
  a1/1 -> Product4/1
  Product8/1 -> Product4/2, Delay4/1
  2K(V+1)/1 -> Product6/1
  a2/1 -> Unary Minus/1
  Sum8/1 -> Product3/2
  Product7/1 -> Product1/2, Delay2/1
  K²(V²+2V+1)+1/1 -> Sum8/1, Sum6/2
  Product5/1 -> Sum2/2
  Delay3/1 -> Product8/1

== system shelf_cascade/Subsystem16/Subsystem8 ==
  DataIn : Inport
  1/a0 : Inport  Port=2
  a1 : Inport  Port=3
  a2 : Inport  Port=4
  2K²(V²+2V+1)-2 : Inport  Port=5
  K²(V²+2V+1)+1 : Inport  Port=6
  2K(V+1) : Inport  Port=7
  Cm : Inport  Port=8
  Enable : EnablePort
  Delay{1..4} (4 alike) : Delay  DelayLength=1  InitialCondition=0
  Product{1..8} (8 alike) : Product  OutDataTypeStr=fixdt(1,27,23)
  Sum1 : Sum  Inputs=|+++
  Sum2 : Sum  Inputs=|++
  Sum4 : Sum  Inputs=|++
  Sum6 : Sum  Inputs=|++
  Sum8 : Sum  Inputs=|+-
  Unary Minus : UnaryMinus
  Unary Minus1 : UnaryMinus
  DataOut : Outport  VectorParamsAs1DForOutWhenUnconnected=off
  wires:
  K²(V²+2V+1)+1/1 -> Sum8/1, Sum6/2
  Product1/1 -> Sum4/1
  Cm/1 -> Product6/2
  Sum1/1 -> Sum4/2
  Delay2/1 -> Product2/1, Delay1/1
  Delay1/1 -> Product3/1
  2K(V+1)/1 -> Product6/1
  Product8/1 -> Product4/2, Delay4/1
  Sum6/1 -> Product1/1
  Product6/1 -> Sum6/1, Sum8/2  "2KCm(V+1)"
  Product7/1 -> Product1/2, Delay2/1
  Unary Minus1/1 -> Product4/1
  2K²(V²+2V+1)-2/1 -> Product2/2
  Unary Minus/1 -> Product5/2
  Sum2/1 -> Sum1/2
  Product4/1 -> Sum1/3
  1/a0/1 -> Product8/2, Product7/2
  Product5/1 -> Sum2/2
  Sum4/1 -> DataOut/1, Delay3/1
  a2/1 -> Unary Minus/1
  Delay3/1 -> Product8/1
  DataIn/1 -> Product7/1
  Product3/1 -> Sum2/1
  Product2/1 -> Sum1/1
  Sum8/1 -> Product3/2
  a1/1 -> Unary Minus1/1
  Delay4/1 -> Product5/1

== system shelf_cascade/Subsystem16/Subsystem9 ==
  K : Inport
  V : Inport  Port=2
  Constant10 : Constant  OutDataTypeStr=fixdt(1,27,23)  SampleTime=-1
  Constant{6,8,11,13} (4 alike) : Constant  Value=2  OutDataTypeStr=fixdt(1,27,23)  SampleTime=-1
  Constant7 : Constant  OutDataTypeStr=fixdt(1,27,23)  SampleTime=-1
  Constant9 : Constant  OutDataTypeStr=fixdt(1,27,23)  SampleTime=-1
  Product{,6..11} (7 alike) : Product  OutDataTypeStr=fixdt(1,27,23)
  Sum3 : Sum  Inputs=|++
  Sum5 : Sum  Inputs=|+++
  Sum6 : Sum  Inputs=|++
  Sum7 : Sum  Inputs=|+-
  2K²(V²+2V+1)-2 : Outport
  K²(V²+2V+1)+1 : Outport  Port=2
  2K(V+1) : Outport  Port=3
  wires:
  Sum7/1 -> 2K²(V²+2V+1)-2/1  "2K²(V²+2V+1)-2"
  K/1 -> Product6/1, Product/2, Product/1  "K"
  Product6/1 -> Product7/1  "2K"
  Product10/1 -> Sum6/1, Product11/1  "K²(V²+2V+1)"
  Product11/1 -> Sum7/1  "2K²(V²+2V+1)"
  Constant7/1 -> Sum3/1
  Constant11/1 -> Sum7/2
  Sum3/1 -> Product7/2  "V+1"
  Product7/1 -> 2K(V+1)/1  "2K(V+1)"
  Constant10/1 -> Sum6/2
  V/1 -> Product9/1, Product8/2, Product8/1, Sum3/2  "V"
  Constant9/1 -> Sum5/3
  Product/1 -> Product10/1  "K²"
  Sum6/1 -> K²(V²+2V+1)+1/1  "K²(V²+2V+1)+1"
  Constant13/1 -> Product11/2
  Product8/1 -> Sum5/1  "V²"
  Constant6/1 -> Product6/2
  Product9/1 -> Sum5/2  "2V"
  Sum5/1 -> Product10/2  "V²+2V+1"
  Constant8/1 -> Product9/2
